simulink subsystem "Motor"  (R2022a)
settings: Solver=VariableStepAuto  StartTime=0.0  StopTime=10.0  RelTol=1e-3
model mask{Parameter1=YASA P400R}
values from neighbouring files (symbols this model uses):
  eff_trans = 0.96    [ModelScript.m]
  ratio_fd = ratio_fd.*0.95    [ModelScript.m]
undefined symbols (not defined in the file or in its folder): eff, EM_Efficiency, EM_Omega_Map, EM_Torque_Map, plant, RPM, Torque, w
settings Model: Creator=HP  LastModifiedBy=saumi

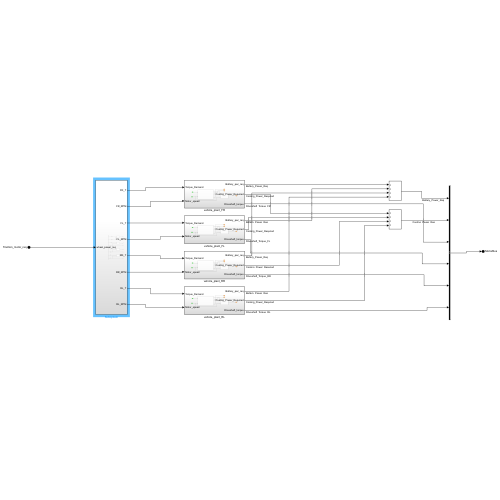
[thumbnail: Simulink's stored preview of the top-level diagram]
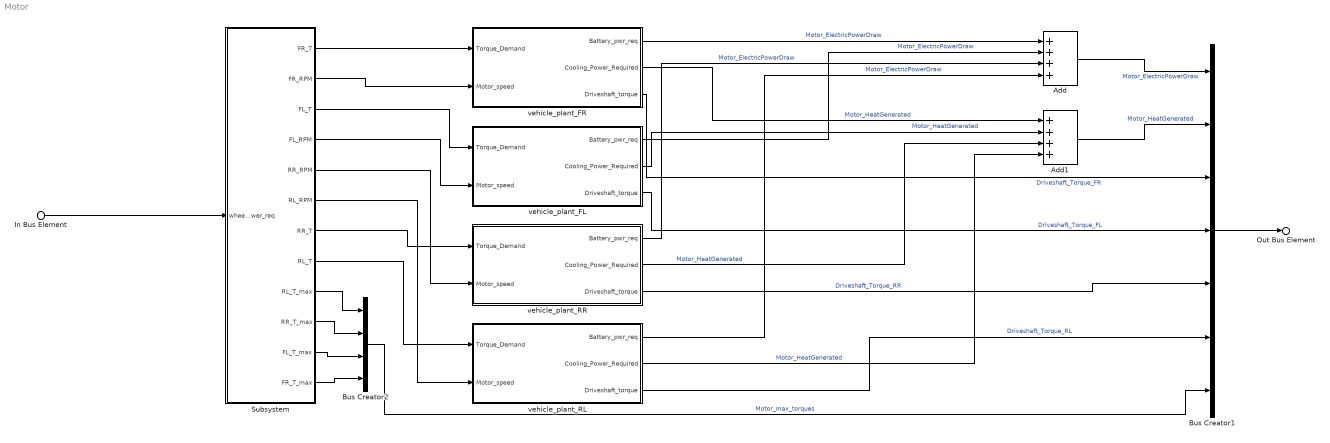
== system Motor ==
  In Bus Element : Inport  PortName=Traction_motor_req
  Add : Sum  Inputs=++++
  Add1 : Sum  Inputs=++++
  Bus Creator1 : BusCreator  Inputs=7
  Bus Creator2 : BusCreator  Inputs=4
  Subsystem : Subsystem
  vehicle_plant_FL : Subsystem
  vehicle_plant_FR : Subsystem
  vehicle_plant_RL : Subsystem
  vehicle_plant_RR : Subsystem
  Out Bus Element : Outport  PortName=Motor_States
  wires:
  Bus Creator1/1 -> Out Bus Element/1
  vehicle_plant_FR/1(Battery_pwr_req) -> Add/1  "Motor_ElectricPowerDraw"
  vehicle_plant_FL/1(Battery_pwr_req) -> Add/2  "Motor_ElectricPowerDraw"
  vehicle_plant_RR/1(Battery_pwr_req) -> Add/3  "Motor_ElectricPowerDraw"
  vehicle_plant_RL/1(Battery_pwr_req) -> Add/4  "Motor_ElectricPowerDraw"
  vehicle_plant_FR/2(Cooling_Power_Required) -> Add1/1  "Motor_HeatGenerated"
  vehicle_plant_FL/2(Cooling_Power_Required) -> Add1/2  "Motor_HeatGenerated"
  vehicle_plant_RR/2(Cooling_Power_Required) -> Add1/3  "Motor_HeatGenerated"
  vehicle_plant_RL/2(Cooling_Power_Required) -> Add1/4  "Motor_HeatGenerated"
  Add/1 -> Bus Creator1/1  "Motor_ElectricPowerDraw"
  Add1/1 -> Bus Creator1/2  "Motor_HeatGenerated"
  vehicle_plant_FR/3(Driveshaft_torque) -> Bus Creator1/3  "Driveshaft_Torque_FR"
  vehicle_plant_FL/3(Driveshaft_torque) -> Bus Creator1/4  "Driveshaft_Torque_FL"
  vehicle_plant_RR/3(Driveshaft_torque) -> Bus Creator1/5  "Driveshaft_Torque_RR"
  vehicle_plant_RL/3(Driveshaft_torque) -> Bus Creator1/6  "Driveshaft_Torque_RL"
  Subsystem/1(FR_T) -> vehicle_plant_FR/1(Torque_Demand)
  Subsystem/2(FR_RPM) -> vehicle_plant_FR/2(Motor_speed)
  Subsystem/3(FL_T) -> vehicle_plant_FL/1(Torque_Demand)
  Subsystem/4(FL_RPM) -> vehicle_plant_FL/2(Motor_speed)
  Subsystem/7(RR_T) -> vehicle_plant_RR/1(Torque_Demand)
  Subsystem/5(RR_RPM) -> vehicle_plant_RR/2(Motor_speed)
  Subsystem/8(RL_T) -> vehicle_plant_RL/1(Torque_Demand)
  Subsystem/6(RL_RPM) -> vehicle_plant_RL/2(Motor_speed)
  In Bus Element/1 -> Subsystem/1(wheel_power_req)
  Subsystem/9(RL_T_max) -> Bus Creator2/1
  Subsystem/10(RR_T_max) -> Bus Creator2/2
  Subsystem/11(FL_T_max) -> Bus Creator2/3
  Subsystem/12(FR_T_max) -> Bus Creator2/4
  Bus Creator2/1 -> Bus Creator1/7  "Motor_max_torques"

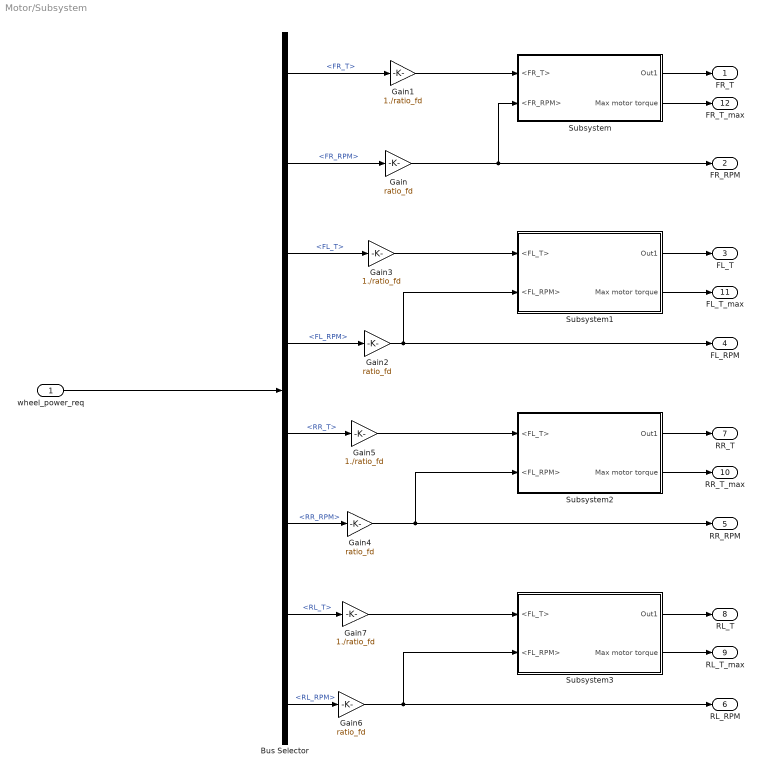
== system Motor/Subsystem ==
  wheel_power_req : Inport
  Bus Selector : BusSelector  OutputSignals=FR_T,FR_RPM,FL_T,FL_RPM,RR_T,RR_RPM,RL_T,RL_RPM
  Gain{,2,4,6} (4 alike) : Gain  Gain=ratio_fd
  Gain{1,3,5,7} (4 alike) : Gain  Gain=1./ratio_fd
  Subsystem : Subsystem
  Subsystem1 : Subsystem
  Subsystem2 : Subsystem
  Subsystem3 : Subsystem
  FR_T : Outport
  FR_RPM : Outport  Port=2
  FL_T : Outport  Port=3
  FL_RPM : Outport  Port=4
  RR_RPM : Outport  Port=5
  RL_RPM : Outport  Port=6
  RR_T : Outport  Port=7
  RL_T : Outport  Port=8
  RL_T_max : Outport  Port=9
  RR_T_max : Outport  Port=10
  FL_T_max : Outport  Port=11
  FR_T_max : Outport  Port=12
  wires:
  Gain7/1 -> Subsystem3/1(<FL_T>)
  Subsystem3/1(Out1) -> RL_T/1
  Gain6/1 -> RL_RPM/1, Subsystem3/2(<FL_RPM>)
  Subsystem3/2(Max motor torque) -> RL_T_max/1
  Gain5/1 -> Subsystem2/1(<FL_T>)
  Subsystem2/1(Out1) -> RR_T/1
  Gain4/1 -> RR_RPM/1, Subsystem2/2(<FL_RPM>)
  Subsystem2/2(Max motor torque) -> RR_T_max/1
  Subsystem1/2(Max motor torque) -> FL_T_max/1
  Subsystem/2(Max motor torque) -> FR_T_max/1
  Bus Selector/2 -> Gain/1  "<FR_RPM>"
  wheel_power_req/1 -> Bus Selector/1
  Bus Selector/1 -> Gain1/1  "<FR_T>"
  Subsystem/1(Out1) -> FR_T/1
  Bus Selector/3 -> Gain3/1  "<FL_T>"
  Bus Selector/4 -> Gain2/1  "<FL_RPM>"
  Subsystem1/1(Out1) -> FL_T/1
  Bus Selector/6 -> Gain4/1  "<RR_RPM>"
  Bus Selector/5 -> Gain5/1  "<RR_T>"
  Bus Selector/7 -> Gain7/1  "<RL_T>"
  Bus Selector/8 -> Gain6/1  "<RL_RPM>"
  Gain/1 -> FR_RPM/1, Subsystem/2(<FR_RPM>)
  Gain1/1 -> Subsystem/1(<FR_T>)
  Gain2/1 -> Subsystem1/2(<FL_RPM>), FL_RPM/1
  Gain3/1 -> Subsystem1/1(<FL_T>)

== system Motor/vehicle_plant_FL ==
  Torque_Demand : Inport
  Motor_speed : Inport  Port=2
  "Traction motor " : Subsystem
  transmission : Subsystem
  Battery_pwr_req : Outport
  Cooling_Power_Required : Outport  Port=2
  Driveshaft_torque : Outport  Port=3
  wires:
  transmission/1(driveshaft_torque) -> Driveshaft_torque/1  "driveshaft_torque"
  Motor_speed/1 -> "Traction motor "/2(motor_speed), transmission/2(motor_speed)
  Torque_Demand/1 -> "Traction motor "/1(Torque_Demand)
  "Traction motor "/1(EM Tq Out) -> transmission/1(motor_torque)  "motor_torque"
  "Traction motor "/3(Batt power) -> Battery_pwr_req/1
  "Traction motor "/2(EM cooling pwr req) -> Cooling_Power_Required/1

== system Motor/vehicle_plant_FR ==
  Torque_Demand : Inport
  Motor_speed : Inport  Port=2
  "Traction motor " : Subsystem
  transmission : Subsystem
  Battery_pwr_req : Outport
  Cooling_Power_Required : Outport  Port=2
  Driveshaft_torque : Outport  Port=3
  wires:
  "Traction motor "/2(EM cooling pwr req) -> Cooling_Power_Required/1
  "Traction motor "/3(Batt power) -> Battery_pwr_req/1
  "Traction motor "/1(EM Tq Out) -> transmission/1(motor_torque)  "motor_torque"
  Torque_Demand/1 -> "Traction motor "/1(Torque_Demand)
  Motor_speed/1 -> transmission/2(motor_speed), "Traction motor "/2(motor_speed)
  transmission/1(driveshaft_torque) -> Driveshaft_torque/1  "driveshaft_torque"

== system Motor/vehicle_plant_RL ==
  Torque_Demand : Inport
  Motor_speed : Inport  Port=2
  "Traction motor " : Subsystem
  transmission : Subsystem
  Battery_pwr_req : Outport
  Cooling_Power_Required : Outport  Port=2
  Driveshaft_torque : Outport  Port=3
  wires:
  "Traction motor "/2(EM cooling pwr req) -> Cooling_Power_Required/1
  "Traction motor "/3(Batt power) -> Battery_pwr_req/1
  "Traction motor "/1(EM Tq Out) -> transmission/1(motor_torque)  "motor_torque"
  Torque_Demand/1 -> "Traction motor "/1(Torque_Demand)
  Motor_speed/1 -> transmission/2(motor_speed), "Traction motor "/2(motor_speed)
  transmission/1(driveshaft_torque) -> Driveshaft_torque/1  "driveshaft_torque"

== system Motor/vehicle_plant_RR ==
  Torque_Demand : Inport
  Motor_speed : Inport  Port=2
  "Traction motor " : Subsystem
  transmission : Subsystem
  Battery_pwr_req : Outport
  Cooling_Power_Required : Outport  Port=2
  Driveshaft_torque : Outport  Port=3
  wires:
  "Traction motor "/2(EM cooling pwr req) -> Cooling_Power_Required/1
  "Traction motor "/3(Batt power) -> Battery_pwr_req/1
  "Traction motor "/1(EM Tq Out) -> transmission/1(motor_torque)  "motor_torque"
  Torque_Demand/1 -> "Traction motor "/1(Torque_Demand)
  Motor_speed/1 -> transmission/2(motor_speed), "Traction motor "/2(motor_speed)
  transmission/1(driveshaft_torque) -> Driveshaft_torque/1  "driveshaft_torque"

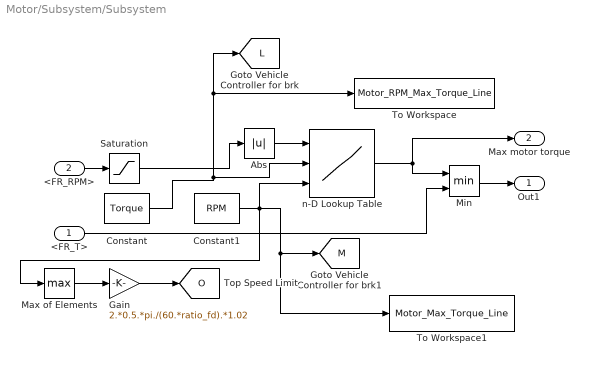
== system Motor/Subsystem/Subsystem ==
  <FR_T> : Inport
  <FR_RPM> : Inport  Port=2
  Abs : Abs  SaturateOnIntegerOverflow=off
  Constant : Constant  Value=Torque
  Constant1 : Constant  Value=RPM
  Gain : Gain  Gain=2.*0.5.*pi./(60.*ratio_fd).*1.02
  Max of Elements : MinMax  Function=max
  Min : MinMax  Inputs=2
  Saturation : Saturate  UpperLimit=max(RPM)  LowerLimit=0
  To Workspace : ToWorkspace  VariableName=Motor_RPM_Max_Torque_Line  SampleTime=-1
      settings: Save2DSignal=2-D array (concatenate along first dimension)
  To Workspace1 : ToWorkspace  VariableName=Motor_Max_Torque_Line  SampleTime=-1
      settings: Save2DSignal=2-D array (concatenate along first dimension)
  n-D Lookup Table : Lookup_n-D  NumberOfTableDimensions=1  LookupTableObject=''  BreakpointsForDimension1Source=Input port  BreakpointsForDimension1=[1:2]  BreakpointsForDimension2Source=Input port  BreakpointsForDimension2=[1:2]  BreakpointsForDimension3Source=Input port  BreakpointsForDimension3=[5, 7]  BreakpointsForDimension1FirstPoint=10  BreakpointsForDimension2FirstPoint=10  BreakpointsForDimension1Spacing=12  BreakpointsForDimension2Spacing=12  IndexSearchMethod=Evenly spaced points  TableSource=Input port  Table=[4 5;16 19]  ExtrapMethod=Clip  DiagnosticForOutOfRangeInput=Warning  UseLastTableValue=on  InternalRulePriority=Speed  RndMeth=Simplest
      settings: InputPortMap=u0,p221,p5
  Out1 : Outport
  Max motor torque : Outport  Port=2
  tag scope: L=global, M=global, O=global
  wires:
  Gain/1 -> [O]
  Max of Elements/1 -> Gain/1
  Constant1/1 -> Max of Elements/1, n-D Lookup Table/3, [M], To Workspace1/1
  Min/1 -> Out1/1
  n-D Lookup Table/1 -> Max motor torque/1, Min/1
  <FR_T>/1 -> Min/2
  Constant/1 -> n-D Lookup Table/2, To Workspace/1, [L]
  Abs/1 -> n-D Lookup Table/1
  <FR_RPM>/1 -> Saturation/1
  Saturation/1 -> Abs/1

== system Motor/Subsystem/Subsystem1 ==
  <FL_T> : Inport
  <FL_RPM> : Inport  Port=2
  Abs : Abs  SaturateOnIntegerOverflow=off
  Constant : Constant  Value=Torque
  Constant1 : Constant  Value=RPM
  Min : MinMax  Inputs=2
  Saturation : Saturate  UpperLimit=max(RPM)  LowerLimit=0
  n-D Lookup Table : Lookup_n-D  NumberOfTableDimensions=1  LookupTableObject=''  BreakpointsForDimension1Source=Input port  BreakpointsForDimension1=[1:2]  BreakpointsForDimension2Source=Input port  BreakpointsForDimension2=[1:2]  BreakpointsForDimension3Source=Input port  BreakpointsForDimension3=[5, 7]  BreakpointsForDimension1FirstPoint=10  BreakpointsForDimension2FirstPoint=10  BreakpointsForDimension1Spacing=12  BreakpointsForDimension2Spacing=12  IndexSearchMethod=Evenly spaced points  TableSource=Input port  Table=[4 5;16 19]  DiagnosticForOutOfRangeInput=Warning  InternalRulePriority=Speed  RndMeth=Simplest
      settings: InputPortMap=u0,p221,p5
  Out1 : Outport
  Max motor torque : Outport  Port=2
  wires:
  n-D Lookup Table/1 -> Max motor torque/1, Min/1
  Constant1/1 -> n-D Lookup Table/3
  Constant/1 -> n-D Lookup Table/2
  Min/1 -> Out1/1
  <FL_RPM>/1 -> Saturation/1
  <FL_T>/1 -> Min/2
  Abs/1 -> n-D Lookup Table/1
  Saturation/1 -> Abs/1

== system Motor/Subsystem/Subsystem2 ==
  <FL_T> : Inport
  <FL_RPM> : Inport  Port=2
  Abs : Abs  SaturateOnIntegerOverflow=off
  Constant : Constant  Value=Torque
  Constant1 : Constant  Value=RPM
  Min : MinMax  Inputs=2
  Saturation : Saturate  UpperLimit=max(RPM)  LowerLimit=0
  n-D Lookup Table : Lookup_n-D  NumberOfTableDimensions=1  LookupTableObject=''  BreakpointsForDimension1Source=Input port  BreakpointsForDimension1=[1:2]  BreakpointsForDimension2Source=Input port  BreakpointsForDimension2=[1:2]  BreakpointsForDimension3Source=Input port  BreakpointsForDimension3=[5, 7]  BreakpointsForDimension1FirstPoint=10  BreakpointsForDimension2FirstPoint=10  BreakpointsForDimension1Spacing=12  BreakpointsForDimension2Spacing=12  IndexSearchMethod=Evenly spaced points  TableSource=Input port  Table=[4 5;16 19]  DiagnosticForOutOfRangeInput=Warning  InternalRulePriority=Speed  RndMeth=Simplest
      settings: InputPortMap=u0,p221,p5
  Out1 : Outport
  Max motor torque : Outport  Port=2
  wires:
  n-D Lookup Table/1 -> Max motor torque/1, Min/1
  Constant1/1 -> n-D Lookup Table/3
  Constant/1 -> n-D Lookup Table/2
  Min/1 -> Out1/1
  <FL_RPM>/1 -> Saturation/1
  <FL_T>/1 -> Min/2
  Abs/1 -> n-D Lookup Table/1
  Saturation/1 -> Abs/1

== system Motor/Subsystem/Subsystem3 ==
  <FL_T> : Inport
  <FL_RPM> : Inport  Port=2
  Abs : Abs  SaturateOnIntegerOverflow=off
  Constant : Constant  Value=Torque
  Constant1 : Constant  Value=RPM
  Min : MinMax  Inputs=2
  Saturation : Saturate  UpperLimit=max(RPM)  LowerLimit=0
  n-D Lookup Table : Lookup_n-D  NumberOfTableDimensions=1  LookupTableObject=''  BreakpointsForDimension1Source=Input port  BreakpointsForDimension1=[1:2]  BreakpointsForDimension2Source=Input port  BreakpointsForDimension2=[1:2]  BreakpointsForDimension3Source=Input port  BreakpointsForDimension3=[5, 7]  BreakpointsForDimension1FirstPoint=10  BreakpointsForDimension2FirstPoint=10  BreakpointsForDimension1Spacing=12  BreakpointsForDimension2Spacing=12  IndexSearchMethod=Evenly spaced points  TableSource=Input port  Table=[4 5;16 19]  DiagnosticForOutOfRangeInput=Warning  InternalRulePriority=Speed  RndMeth=Simplest
      settings: InputPortMap=u0,p221,p5
  Out1 : Outport
  Max motor torque : Outport  Port=2
  wires:
  n-D Lookup Table/1 -> Max motor torque/1, Min/1
  Constant1/1 -> n-D Lookup Table/3
  Constant/1 -> n-D Lookup Table/2
  Min/1 -> Out1/1
  <FL_RPM>/1 -> Saturation/1
  <FL_T>/1 -> Min/2
  Abs/1 -> n-D Lookup Table/1
  Saturation/1 -> Abs/1

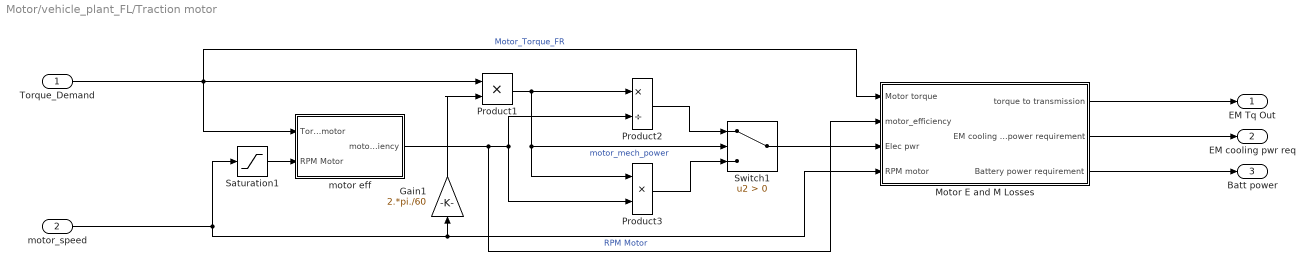
== system Motor/vehicle_plant_FL/Traction motor  ==
  Torque_Demand : Inport
  motor_speed : Inport  Port=2
  Gain1 : Gain  Gain=2.*pi./60
  Motor E and M Losses : Subsystem
  Product1 : Product
  Product2 : Product  Inputs=*/
  Product3 : Product  Inputs=**
  Saturation1 : Saturate  UpperLimit=8000  LowerLimit=-8000
  Switch1 : Switch  Criteria=u2 > Threshold  SaturateOnIntegerOverflow=off  InputSameDT=off
  motor eff : Subsystem
  EM Tq Out : Outport
  EM cooling pwr req : Outport  Port=2
  Batt power : Outport  Port=3
  wires:
  Product1/1 -> Product3/1, Switch1/2, Product2/1  "motor_mech_power"
  Product2/1 -> Switch1/1
  Product3/1 -> Switch1/3
  Switch1/1 -> Motor E and M Losses/3(Elec pwr)
  motor_speed/1 -> Saturation1/1, Gain1/1, Motor E and M Losses/4(RPM motor)  "RPM Motor"
  Motor E and M Losses/1(torque to transmission) -> EM Tq Out/1
  Motor E and M Losses/2(EM cooling power requirement) -> EM cooling pwr req/1
  Motor E and M Losses/3(Battery power requirement) -> Batt power/1
  motor eff/1(motor_efficiency) -> Product3/2, Product2/2, Motor E and M Losses/2(motor_efficiency)
  Saturation1/1 -> motor eff/2(RPM Motor)
  Gain1/1 -> Product1/2
  Torque_Demand/1 -> motor eff/1(Torque motor), Product1/1, Motor E and M Losses/1(Motor torque)  "Motor_Torque_FR"

== system Motor/vehicle_plant_FL/transmission ==
  motor_torque : Inport
  motor_speed : Inport  Port=2
  Gain : Gain  Gain=ratio_fd
  Power flow from motor to driveshaft : Gain  Gain=eff_trans
  Product : Product
  Switch : Switch  Criteria=u2 > Threshold  ZeroCross=off  SaturateOnIntegerOverflow=off  InputSameDT=off
  driveshaft to motor : Gain  Gain=1/eff_trans
  driveshaft_torque : Outport
  wires:
  motor_speed/1 -> Product/2
  motor_torque/1 -> Power flow from motor to driveshaft/1, Product/1, driveshaft to motor/1
  Switch/1 -> Gain/1
  driveshaft to motor/1 -> Switch/3
  Power flow from motor to driveshaft/1 -> Switch/1
  Gain/1 -> driveshaft_torque/1
  Product/1 -> Switch/2

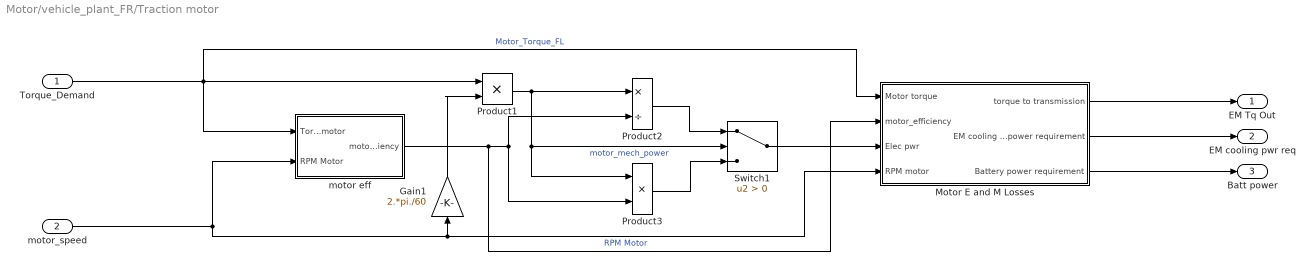
== system Motor/vehicle_plant_FR/Traction motor  ==
  Torque_Demand : Inport
  motor_speed : Inport  Port=2
  Gain1 : Gain  Gain=2.*pi./60
  Motor E and M Losses : Subsystem
  Product1 : Product
  Product2 : Product  Inputs=*/
  Product3 : Product  Inputs=**
  Switch1 : Switch  Criteria=u2 > Threshold  SaturateOnIntegerOverflow=off  InputSameDT=off
  motor eff : Subsystem
  EM Tq Out : Outport
  EM cooling pwr req : Outport  Port=2
  Batt power : Outport  Port=3
  wires:
  Torque_Demand/1 -> Motor E and M Losses/1(Motor torque), Product1/1, motor eff/1(Torque motor)  "Motor_Torque_FL"
  Gain1/1 -> Product1/2
  motor eff/1(motor_efficiency) -> Motor E and M Losses/2(motor_efficiency), Product2/2, Product3/2
  Motor E and M Losses/3(Battery power requirement) -> Batt power/1
  Motor E and M Losses/2(EM cooling power requirement) -> EM cooling pwr req/1
  Motor E and M Losses/1(torque to transmission) -> EM Tq Out/1
  motor_speed/1 -> Motor E and M Losses/4(RPM motor), Gain1/1, motor eff/2(RPM Motor)  "RPM Motor"
  Switch1/1 -> Motor E and M Losses/3(Elec pwr)
  Product3/1 -> Switch1/3
  Product2/1 -> Switch1/1
  Product1/1 -> Product2/1, Switch1/2, Product3/1  "motor_mech_power"

== system Motor/vehicle_plant_FR/transmission ==
  motor_torque : Inport
  motor_speed : Inport  Port=2
  Gain : Gain  Gain=ratio_fd
  Power flow from motor to driveshaft : Gain  Gain=eff_trans
  Product : Product
  Switch : Switch  Criteria=u2 > Threshold  ZeroCross=off  SaturateOnIntegerOverflow=off  InputSameDT=off
  driveshaft to motor : Gain  Gain=1/eff_trans
  driveshaft_torque : Outport
  wires:
  Product/1 -> Switch/2
  Gain/1 -> driveshaft_torque/1
  Power flow from motor to driveshaft/1 -> Switch/1
  driveshaft to motor/1 -> Switch/3
  Switch/1 -> Gain/1
  motor_torque/1 -> driveshaft to motor/1, Product/1, Power flow from motor to driveshaft/1
  motor_speed/1 -> Product/2

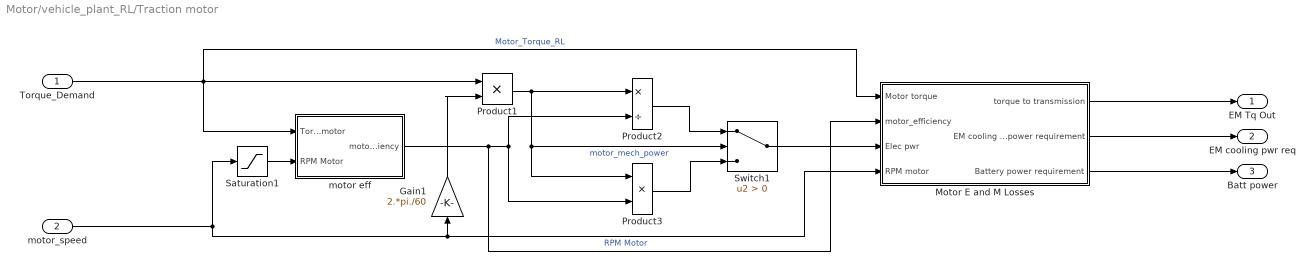
== system Motor/vehicle_plant_RL/Traction motor  ==
  Torque_Demand : Inport
  motor_speed : Inport  Port=2
  Gain1 : Gain  Gain=2.*pi./60
  Motor E and M Losses : Subsystem
  Product1 : Product
  Product2 : Product  Inputs=*/
  Product3 : Product  Inputs=**
  Saturation1 : Saturate  UpperLimit=8000  LowerLimit=-8000
  Switch1 : Switch  Criteria=u2 > Threshold  SaturateOnIntegerOverflow=off  InputSameDT=off
  motor eff : Subsystem
  EM Tq Out : Outport
  EM cooling pwr req : Outport  Port=2
  Batt power : Outport  Port=3
  wires:
  Torque_Demand/1 -> Motor E and M Losses/1(Motor torque), Product1/1, motor eff/1(Torque motor)  "Motor_Torque_RL"
  Gain1/1 -> Product1/2
  Saturation1/1 -> motor eff/2(RPM Motor)
  motor eff/1(motor_efficiency) -> Motor E and M Losses/2(motor_efficiency), Product2/2, Product3/2
  Motor E and M Losses/3(Battery power requirement) -> Batt power/1
  Motor E and M Losses/2(EM cooling power requirement) -> EM cooling pwr req/1
  Motor E and M Losses/1(torque to transmission) -> EM Tq Out/1
  motor_speed/1 -> Motor E and M Losses/4(RPM motor), Gain1/1, Saturation1/1  "RPM Motor"
  Switch1/1 -> Motor E and M Losses/3(Elec pwr)
  Product3/1 -> Switch1/3
  Product2/1 -> Switch1/1
  Product1/1 -> Product2/1, Switch1/2, Product3/1  "motor_mech_power"

== system Motor/vehicle_plant_RL/transmission ==
  motor_torque : Inport
  motor_speed : Inport  Port=2
  Gain : Gain  Gain=ratio_fd
  Power flow from motor to driveshaft : Gain  Gain=eff_trans
  Product : Product
  Switch : Switch  Criteria=u2 > Threshold  ZeroCross=off  SaturateOnIntegerOverflow=off  InputSameDT=off
  driveshaft to motor : Gain  Gain=1/eff_trans
  driveshaft_torque : Outport
  wires:
  Product/1 -> Switch/2
  Gain/1 -> driveshaft_torque/1
  Power flow from motor to driveshaft/1 -> Switch/1
  driveshaft to motor/1 -> Switch/3
  Switch/1 -> Gain/1
  motor_torque/1 -> driveshaft to motor/1, Product/1, Power flow from motor to driveshaft/1
  motor_speed/1 -> Product/2

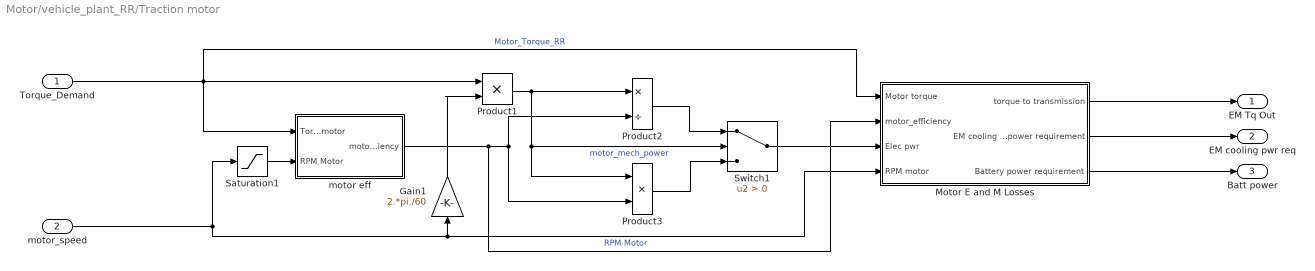
== system Motor/vehicle_plant_RR/Traction motor  ==
  Torque_Demand : Inport
  motor_speed : Inport  Port=2
  Gain1 : Gain  Gain=2.*pi./60
  Motor E and M Losses : Subsystem
  Product1 : Product
  Product2 : Product  Inputs=*/
  Product3 : Product  Inputs=**
  Saturation1 : Saturate  UpperLimit=8000  LowerLimit=-8000
  Switch1 : Switch  Criteria=u2 > Threshold  SaturateOnIntegerOverflow=off  InputSameDT=off
  motor eff : Subsystem
  EM Tq Out : Outport
  EM cooling pwr req : Outport  Port=2
  Batt power : Outport  Port=3
  wires:
  Torque_Demand/1 -> Motor E and M Losses/1(Motor torque), Product1/1, motor eff/1(Torque motor)  "Motor_Torque_RR"
  Gain1/1 -> Product1/2
  Saturation1/1 -> motor eff/2(RPM Motor)
  motor eff/1(motor_efficiency) -> Motor E and M Losses/2(motor_efficiency), Product2/2, Product3/2
  Motor E and M Losses/3(Battery power requirement) -> Batt power/1
  Motor E and M Losses/2(EM cooling power requirement) -> EM cooling pwr req/1
  Motor E and M Losses/1(torque to transmission) -> EM Tq Out/1
  motor_speed/1 -> Motor E and M Losses/4(RPM motor), Gain1/1, Saturation1/1  "RPM Motor"
  Switch1/1 -> Motor E and M Losses/3(Elec pwr)
  Product3/1 -> Switch1/3
  Product2/1 -> Switch1/1
  Product1/1 -> Product2/1, Switch1/2, Product3/1  "motor_mech_power"

== system Motor/vehicle_plant_RR/transmission ==
  motor_torque : Inport
  motor_speed : Inport  Port=2
  Gain : Gain  Gain=ratio_fd
  Power flow from motor to driveshaft : Gain  Gain=eff_trans
  Product : Product
  Switch : Switch  Criteria=u2 > Threshold  ZeroCross=off  SaturateOnIntegerOverflow=off  InputSameDT=off
  driveshaft to motor : Gain  Gain=1/eff_trans
  driveshaft_torque : Outport
  wires:
  Product/1 -> Switch/2
  Gain/1 -> driveshaft_torque/1
  Power flow from motor to driveshaft/1 -> Switch/1
  driveshaft to motor/1 -> Switch/3
  Switch/1 -> Gain/1
  motor_torque/1 -> driveshaft to motor/1, Product/1, Power flow from motor to driveshaft/1
  motor_speed/1 -> Product/2

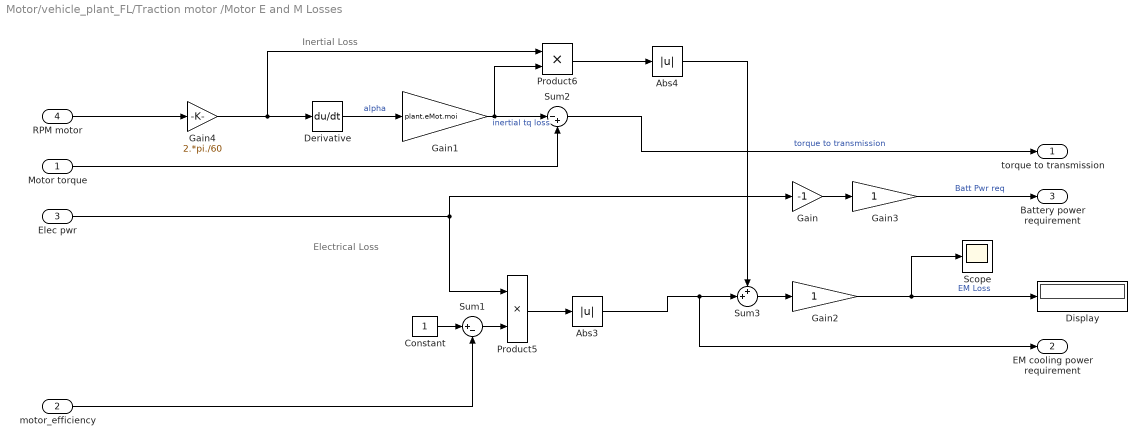
== system Motor/vehicle_plant_FL/Traction motor /Motor E and M Losses ==
  note: Electrical Loss
  note: Inertial Loss
  Motor torque : Inport
  motor_efficiency : Inport  Port=2
  Elec pwr : Inport  Port=3
  RPM motor : Inport  Port=4
  Abs3 : Abs  SaturateOnIntegerOverflow=off
  Abs4 : Abs  ZeroCross=off  SaturateOnIntegerOverflow=off
  Constant : Constant
  Derivative : Derivative
  Display : Display
  Gain : Gain  Gain=-1
  Gain1 : Gain  Gain=plant.eMot.moi
  Gain2 : Gain
  Gain3 : Gain
  Gain4 : Gain  Gain=2.*pi./60
  Product5 : Product
  Product6 : Product
  Scope : Scope
  Sum1 : Sum  Inputs=|+-
  Sum2 : Sum  Inputs=|-+
  Sum3 : Sum  Inputs=++|
  torque to transmission : Outport
  EM cooling power requirement : Outport  Port=2
  Battery power requirement : Outport  Port=3
  wires:
  Gain4/1 -> Product6/1, Derivative/1
  Motor torque/1 -> Sum2/2
  RPM motor/1 -> Gain4/1
  Elec pwr/1 -> Gain/1, Product5/1
  Abs3/1 -> EM cooling power requirement/1, Sum3/2
  Sum3/1 -> Gain2/1
  Sum1/1 -> Product5/2
  Gain2/1 -> Display/1, Scope/1  "EM Loss"
  Product5/1 -> Abs3/1
  Gain1/1 -> Product6/2, Sum2/1  "inertial tq loss"
  Abs4/1 -> Sum3/1
  Constant/1 -> Sum1/1
  Product6/1 -> Abs4/1
  Derivative/1 -> Gain1/1  "alpha"
  Sum2/1 -> torque to transmission/1  "torque to transmission"
  motor_efficiency/1 -> Sum1/2
  Gain/1 -> Gain3/1
  Gain3/1 -> Battery power requirement/1  "Batt Pwr req"

== system Motor/vehicle_plant_FL/Traction motor /motor eff ==
  Torque motor : Inport
  RPM Motor : Inport  Port=2
  Abs1 : Abs  SaturateOnIntegerOverflow=off
  Abs2 : Abs  SaturateOnIntegerOverflow=off
  Constant : Constant  Value=eff
  Constant1 : Constant  Value=t
  Constant2 : Constant  Value=w
  Motor efficency map : Lookup_n-D  BreakpointsForDimension1Source=Input port  BreakpointsForDimension1=EM_Torque_Map  BreakpointsForDimension2Source=Input port  BreakpointsForDimension2=EM_Omega_Map  TableSource=Input port  Table=EM_Efficiency  ExtrapMethod=Clip  InternalRulePriority=Speed  RndMeth=Simplest
      settings: InputPortMap=u0,u1,p221,p5,p7
  motor_efficiency : Outport
  wires:
  Constant2/1 -> Motor efficency map/5  "RPM"
  Constant1/1 -> Motor efficency map/4  "Torque"
  Constant/1 -> Motor efficency map/3  "Eff"
  Torque motor/1 -> Abs1/1
  Motor efficency map/1 -> motor_efficiency/1  "motor_efficiency"
  RPM Motor/1 -> Abs2/1
  Abs2/1 -> Motor efficency map/2
  Abs1/1 -> Motor efficency map/1

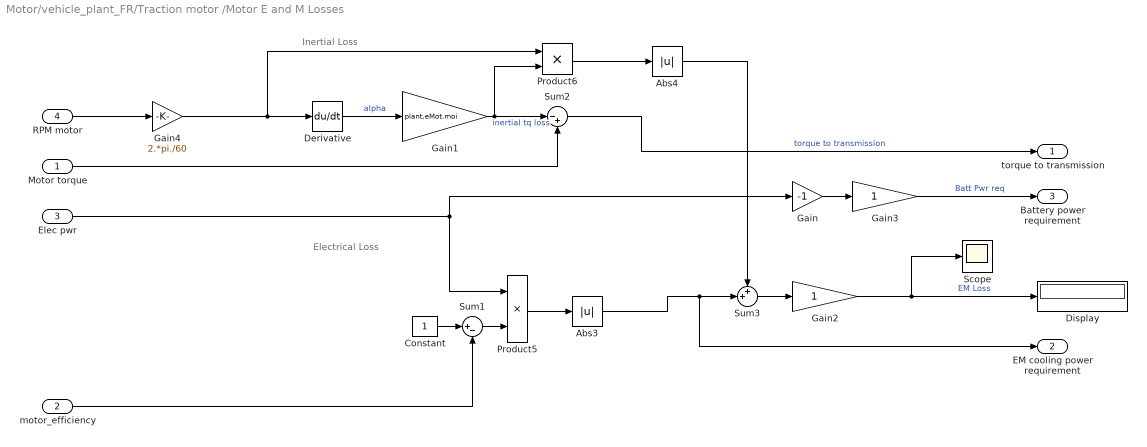
== system Motor/vehicle_plant_FR/Traction motor /Motor E and M Losses ==
  note: Inertial Loss
  note: Electrical Loss
  Motor torque : Inport
  motor_efficiency : Inport  Port=2
  Elec pwr : Inport  Port=3
  RPM motor : Inport  Port=4
  Abs3 : Abs  SaturateOnIntegerOverflow=off
  Abs4 : Abs  ZeroCross=off  SaturateOnIntegerOverflow=off
  Constant : Constant
  Derivative : Derivative
  Display : Display
  Gain : Gain  Gain=-1
  Gain1 : Gain  Gain=plant.eMot.moi
  Gain2 : Gain
  Gain3 : Gain
  Gain4 : Gain  Gain=2.*pi./60
  Product5 : Product
  Product6 : Product
  Scope : Scope
  Sum1 : Sum  Inputs=|+-
  Sum2 : Sum  Inputs=|-+
  Sum3 : Sum  Inputs=++|
  torque to transmission : Outport
  EM cooling power requirement : Outport  Port=2
  Battery power requirement : Outport  Port=3
  wires:
  Gain4/1 -> Derivative/1, Product6/1
  Gain3/1 -> Battery power requirement/1  "Batt Pwr req"
  Gain/1 -> Gain3/1
  motor_efficiency/1 -> Sum1/2
  Sum2/1 -> torque to transmission/1  "torque to transmission"
  Derivative/1 -> Gain1/1  "alpha"
  Elec pwr/1 -> Product5/1, Gain/1
  Product6/1 -> Abs4/1
  Constant/1 -> Sum1/1
  Abs4/1 -> Sum3/1
  Gain1/1 -> Sum2/1, Product6/2  "inertial tq loss"
  Product5/1 -> Abs3/1
  Gain2/1 -> Scope/1, Display/1  "EM Loss"
  Sum1/1 -> Product5/2
  Sum3/1 -> Gain2/1
  Abs3/1 -> Sum3/2, EM cooling power requirement/1
  RPM motor/1 -> Gain4/1
  Motor torque/1 -> Sum2/2

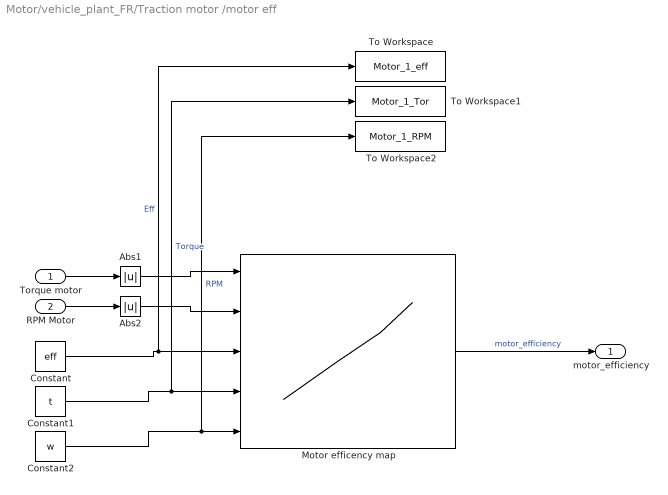
== system Motor/vehicle_plant_FR/Traction motor /motor eff ==
  Torque motor : Inport
  RPM Motor : Inport  Port=2
  Abs1 : Abs  SaturateOnIntegerOverflow=off
  Abs2 : Abs  SaturateOnIntegerOverflow=off
  Constant : Constant  Value=eff
  Constant1 : Constant  Value=t
  Constant2 : Constant  Value=w
  Motor efficency map : Lookup_n-D  BreakpointsForDimension1Source=Input port  BreakpointsForDimension1=EM_Torque_Map  BreakpointsForDimension2Source=Input port  BreakpointsForDimension2=EM_Omega_Map  TableSource=Input port  Table=EM_Efficiency  ExtrapMethod=Clip  InternalRulePriority=Speed  RndMeth=Simplest
      settings: InputPortMap=u0,u1,p221,p5,p7
  To Workspace : ToWorkspace  VariableName=Motor_1_eff  SaveFormat=Timeseries  SampleTime=-1
  To Workspace1 : ToWorkspace  VariableName=Motor_1_Tor  SaveFormat=Timeseries  SampleTime=-1
  To Workspace2 : ToWorkspace  VariableName=Motor_1_RPM  SaveFormat=Timeseries  SampleTime=-1
  motor_efficiency : Outport
  wires:
  Constant2/1 -> To Workspace2/1, Motor efficency map/5  "RPM"
  Constant1/1 -> To Workspace1/1, Motor efficency map/4  "Torque"
  Constant/1 -> To Workspace/1, Motor efficency map/3  "Eff"
  Torque motor/1 -> Abs1/1
  Motor efficency map/1 -> motor_efficiency/1  "motor_efficiency"
  RPM Motor/1 -> Abs2/1
  Abs2/1 -> Motor efficency map/2
  Abs1/1 -> Motor efficency map/1

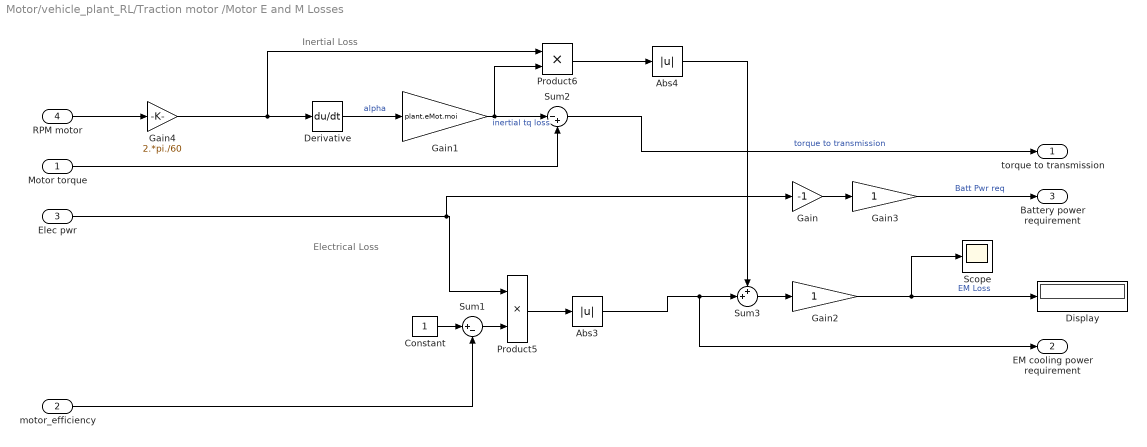
== system Motor/vehicle_plant_RL/Traction motor /Motor E and M Losses ==
  note: Inertial Loss
  note: Electrical Loss
  Motor torque : Inport
  motor_efficiency : Inport  Port=2
  Elec pwr : Inport  Port=3
  RPM motor : Inport  Port=4
  Abs3 : Abs  SaturateOnIntegerOverflow=off
  Abs4 : Abs  ZeroCross=off  SaturateOnIntegerOverflow=off
  Constant : Constant
  Derivative : Derivative
  Display : Display
  Gain : Gain  Gain=-1
  Gain1 : Gain  Gain=plant.eMot.moi
  Gain2 : Gain
  Gain3 : Gain
  Gain4 : Gain  Gain=2.*pi./60
  Product5 : Product
  Product6 : Product
  Scope : Scope
  Sum1 : Sum  Inputs=|+-
  Sum2 : Sum  Inputs=|-+
  Sum3 : Sum  Inputs=++|
  torque to transmission : Outport
  EM cooling power requirement : Outport  Port=2
  Battery power requirement : Outport  Port=3
  wires:
  Gain4/1 -> Derivative/1, Product6/1
  Gain3/1 -> Battery power requirement/1  "Batt Pwr req"
  Gain/1 -> Gain3/1
  motor_efficiency/1 -> Sum1/2
  Sum2/1 -> torque to transmission/1  "torque to transmission"
  Derivative/1 -> Gain1/1  "alpha"
  Product6/1 -> Abs4/1
  Constant/1 -> Sum1/1
  Abs4/1 -> Sum3/1
  Gain1/1 -> Sum2/1, Product6/2  "inertial tq loss"
  Product5/1 -> Abs3/1
  Gain2/1 -> Scope/1, Display/1  "EM Loss"
  Sum1/1 -> Product5/2
  Sum3/1 -> Gain2/1
  Abs3/1 -> Sum3/2, EM cooling power requirement/1
  Elec pwr/1 -> Product5/1, Gain/1
  RPM motor/1 -> Gain4/1
  Motor torque/1 -> Sum2/2

== system Motor/vehicle_plant_RL/Traction motor /motor eff ==
  Torque motor : Inport
  RPM Motor : Inport  Port=2
  Abs1 : Abs  SaturateOnIntegerOverflow=off
  Abs2 : Abs  SaturateOnIntegerOverflow=off
  Constant : Constant  Value=eff
  Constant1 : Constant  Value=t
  Constant2 : Constant  Value=w
  Motor efficency map : Lookup_n-D  BreakpointsForDimension1Source=Input port  BreakpointsForDimension1=EM_Torque_Map  BreakpointsForDimension2Source=Input port  BreakpointsForDimension2=EM_Omega_Map  TableSource=Input port  Table=EM_Efficiency  ExtrapMethod=Clip  InternalRulePriority=Speed  RndMeth=Simplest
      settings: InputPortMap=u0,u1,p221,p5,p7
  motor_efficiency : Outport
  wires:
  Motor efficency map/1 -> motor_efficiency/1  "motor_efficiency"
  Abs2/1 -> Motor efficency map/2
  Constant2/1 -> Motor efficency map/5  "RPM"
  RPM Motor/1 -> Abs2/1
  Abs1/1 -> Motor efficency map/1
  Torque motor/1 -> Abs1/1
  Constant1/1 -> Motor efficency map/4  "Torque"
  Constant/1 -> Motor efficency map/3  "Eff"

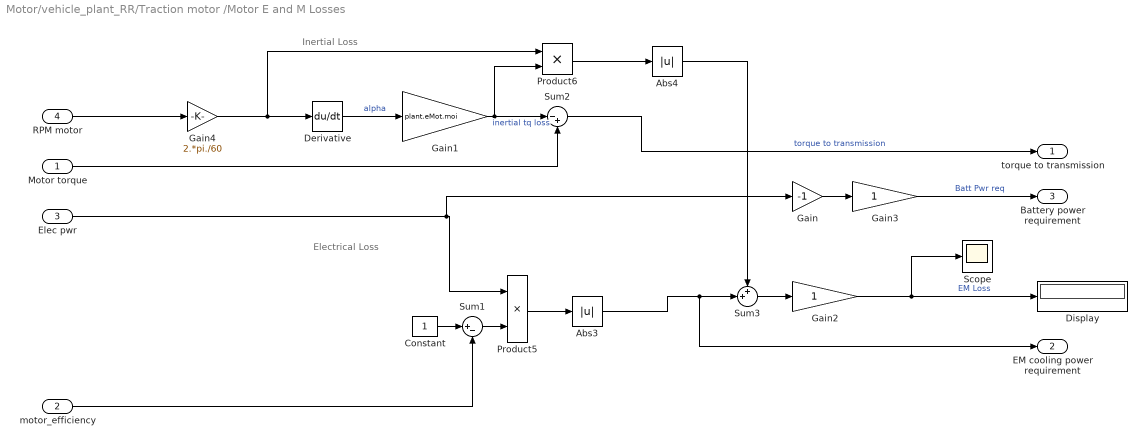
== system Motor/vehicle_plant_RR/Traction motor /Motor E and M Losses ==
  note: Inertial Loss
  note: Electrical Loss
  Motor torque : Inport
  motor_efficiency : Inport  Port=2
  Elec pwr : Inport  Port=3
  RPM motor : Inport  Port=4
  Abs3 : Abs  SaturateOnIntegerOverflow=off
  Abs4 : Abs  ZeroCross=off  SaturateOnIntegerOverflow=off
  Constant : Constant
  Derivative : Derivative
  Display : Display
  Gain : Gain  Gain=-1
  Gain1 : Gain  Gain=plant.eMot.moi
  Gain2 : Gain
  Gain3 : Gain
  Gain4 : Gain  Gain=2.*pi./60
  Product5 : Product
  Product6 : Product
  Scope : Scope
  Sum1 : Sum  Inputs=|+-
  Sum2 : Sum  Inputs=|-+
  Sum3 : Sum  Inputs=++|
  torque to transmission : Outport
  EM cooling power requirement : Outport  Port=2
  Battery power requirement : Outport  Port=3
  wires:
  Gain4/1 -> Derivative/1, Product6/1
  Gain3/1 -> Battery power requirement/1  "Batt Pwr req"
  Gain/1 -> Gain3/1
  motor_efficiency/1 -> Sum1/2
  Sum2/1 -> torque to transmission/1  "torque to transmission"
  Derivative/1 -> Gain1/1  "alpha"
  Product6/1 -> Abs4/1
  Constant/1 -> Sum1/1
  Abs4/1 -> Sum3/1
  Gain1/1 -> Sum2/1, Product6/2  "inertial tq loss"
  Product5/1 -> Abs3/1
  Gain2/1 -> Scope/1, Display/1  "EM Loss"
  Sum1/1 -> Product5/2
  Sum3/1 -> Gain2/1
  Abs3/1 -> Sum3/2, EM cooling power requirement/1
  Elec pwr/1 -> Product5/1, Gain/1
  RPM motor/1 -> Gain4/1
  Motor torque/1 -> Sum2/2

== system Motor/vehicle_plant_RR/Traction motor /motor eff ==
  Torque motor : Inport
  RPM Motor : Inport  Port=2
  Abs1 : Abs  SaturateOnIntegerOverflow=off
  Abs2 : Abs  SaturateOnIntegerOverflow=off
  Constant : Constant  Value=eff
  Constant1 : Constant  Value=t
  Constant2 : Constant  Value=w
  Motor efficency map : Lookup_n-D  BreakpointsForDimension1Source=Input port  BreakpointsForDimension1=EM_Torque_Map  BreakpointsForDimension2Source=Input port  BreakpointsForDimension2=EM_Omega_Map  TableSource=Input port  Table=EM_Efficiency  ExtrapMethod=Clip  InternalRulePriority=Speed  RndMeth=Simplest
      settings: InputPortMap=u0,u1,p221,p5,p7
  motor_efficiency : Outport
  wires:
  Motor efficency map/1 -> motor_efficiency/1  "motor_efficiency"
  Abs2/1 -> Motor efficency map/2
  Constant2/1 -> Motor efficency map/5  "RPM"
  RPM Motor/1 -> Abs2/1
  Abs1/1 -> Motor efficency map/1
  Torque motor/1 -> Abs1/1
  Constant1/1 -> Motor efficency map/4  "Torque"
  Constant/1 -> Motor efficency map/3  "Eff"
